simulink model "Gripper_Wrist_PID_check"  (R2019b)
settings: Solver=VariableStepAuto  StartTime=0.0  StopTime=10.0  FixedStep=0.0001  RelTol=1e-3
undefined symbols (not defined in the file): GR, WB, WJ, WKb, WKm, WL
libraries: cstblocks x2, simulink x1
settings Model: Creator=harsh  LastModifiedBy=harsh

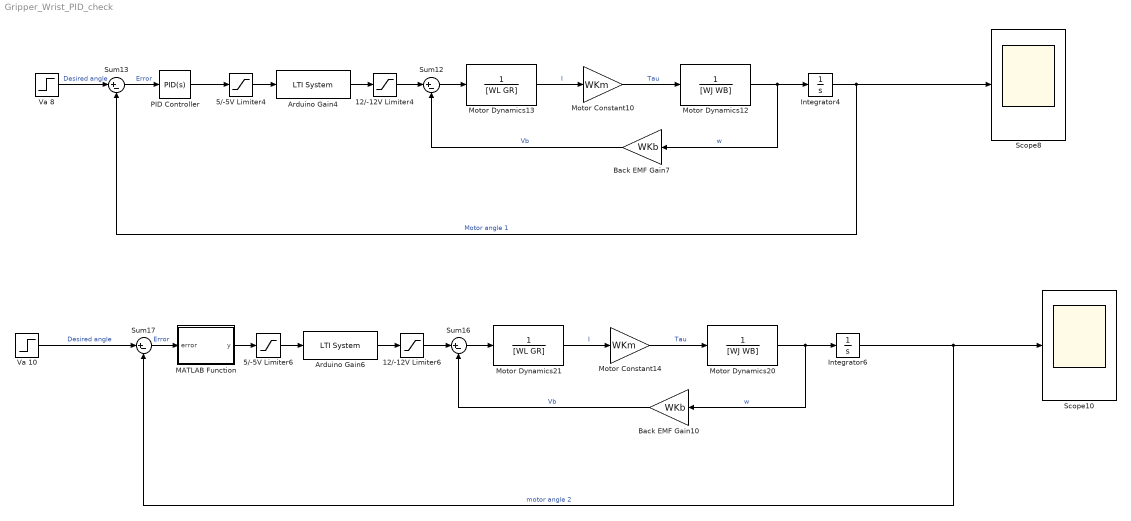
== system Gripper_Wrist_PID_check ==
  12/-12V Limiter4 : Saturate  UpperLimit=12  LowerLimit=-12
  12/-12V Limiter6 : Saturate  UpperLimit=12  LowerLimit=-12
  5/-5V Limiter4 : Saturate  UpperLimit=5  LowerLimit=-5
  5/-5V Limiter6 : Saturate  UpperLimit=5  LowerLimit=-5
  Arduino Gain4 : cstblocks/LTI System  sys=OPAMP  IC=[]
  Arduino Gain6 : cstblocks/LTI System  sys=OPAMP  IC=[]
  Back EMF Gain10 : Gain  Gain=WKb
  Back EMF Gain7 : Gain  Gain=WKb
  Integrator4 : Integrator
  Integrator6 : Integrator
  MATLAB Function : MATLAB Function  TreatAsAtomicUnit=on
  Motor Constant10 : Gain  Gain=WKm
  Motor Constant14 : Gain  Gain=WKm
  Motor Dynamics12 : TransferFcn  Denominator=[WJ WB]
  Motor Dynamics13 : TransferFcn  Denominator=[WL GR]
  Motor Dynamics20 : TransferFcn  Denominator=[WJ WB]
  Motor Dynamics21 : TransferFcn  Denominator=[WL GR]
  PID Controller : simulink/Continuous/PID Controller  Controller=PID  Form=Parallel  TimeDomain=Continuous-time  SampleTime=-1  IntegratorMethod=Forward Euler  FilterMethod=Forward Euler  ControllerParametersSource=internal  P=7.36971279377399  I=24.525158078184  D=0.0474430843490964  UseFilter=on  N=5000  TunerSelectOption=Transfer Function Based (PID Tuner App)  InitialConditionSource=internal  InitialConditionForIntegrator=0  InitialConditionForFilter=0  DifferentiatorICPrevScaledInput=0  ExternalReset=none  TrackingMode=off  Kt=1  LimitOutput=off  UpperSaturationLimit=inf  LowerSaturationLimit=-inf  LinearizeAsGain=on  AntiWindupMode=none  Kb=1  POutMin=[]  POutMax=[]  IOutMin=[]  IOutMax=[]  DOutMin=[]  DOutMax=[]  NOutMin=[]  NOutMax=[]  SumOutMin=[]  SumOutMax=[]  SaturationOutMin=[]  SaturationOutMax=[]  PParamMin=[]  PParamMax=[]  IParamMin=[]  IParamMax=[]  DParamMin=[]  DParamMax=[]  NParamMin=[]  NParamMax=[]  KbParamMin=[]  KbParamMax=[]  KtParamMin=[]  KtParamMax=[]  KbOutMin=[]  KbOutMax=[]  KtOutMin=[]  KtOutMax=[]  IntegratorOutMin=[]  IntegratorOutMax=[]  FilterOutMin=[]  FilterOutMax=[]  SumI1OutMin=[]  SumI1OutMax=[]  SumI2OutMin=[]  SumI2OutMax=[]  SumI3OutMin=[]  SumI3OutMax=[]  SumI4OutMin=[]  SumI4OutMax=[]  SumDOutMin=[]  SumDOutMax=[]  DifferentiatorOutMin=[]  DifferentiatorOutMax=[]  FilterDiffOutCoefMin=[]  FilterDiffOutCoefMax=[]  ReciprocalOutMin=[]  ReciprocalOutMax=[]  SumDenOutMin=[]  SumDenOutMax=[]  SumNumOutMin=[]  SumNumOutMax=[]  DivideOutMin=[]  DivideOutMax=[]  IntegratorContinuousStateAttributes=''  IntegratorStateMustResolveToSignalObject=off  IntegratorRTWStateStorageClass=Auto  FilterContinuousStateAttributes=''  FilterStateMustResolveToSignalObject=off  FilterRTWStateStorageClass=Auto  ParallelPVariant=InternalParameters  IdealPVariant=Disabled  IVariant=InternalParameters  DVariant=InternalParameters  IntegratorVariant=Continuous  SatVariant=Disabled  AWVariant=Passthrough  PCopyVariant=Disabled  TRVariant=Disabled  FdbkBlocksVariant=Forward  IdealPFdbkVariant=Disabled  SatFdbkVariant=Disabled  DerivativeFilterVariant=ContFilter  NVariant=InternalParameters  NCopyVariant=Disabled  FilterICVariant=InternalICsFilter  IntegratorICVariant=InternalICs  ExternalResetVariant=Disabled  TRSumVariant=Passthrough  SumFdbkVariant=Disabled  SumVariant=Sum_PID
  Scope10 : Scope
  Scope8 : Scope
  Sum{12..13,16..17} (4 alike) : Sum  Inputs=|+-
  Va 10 : Step  After=pi/2  SampleTime=0
  Va 8 : Step  After=pi/2  SampleTime=0
  wires:
  Integrator6/1 -> Sum17/2, Scope10/1  "motor angle 2"
  Motor Dynamics20/1 -> Back EMF Gain10/1, Integrator6/1  "w"
  Sum16/1 -> Motor Dynamics21/1
  12/-12V Limiter6/1 -> Sum16/1
  Motor Constant14/1 -> Motor Dynamics20/1  "Tau"
  Sum17/1 -> MATLAB Function/1(error)  "Error"
  Motor Dynamics21/1 -> Motor Constant14/1  "I"
  5/-5V Limiter4/1 -> Arduino Gain4/1
  Back EMF Gain10/1 -> Sum16/2  "Vb"
  Arduino Gain4/1 -> 12/-12V Limiter4/1
  Back EMF Gain7/1 -> Sum12/2  "Vb"
  Integrator4/1 -> Scope8/1, Sum13/2  "Motor angle 1"
  5/-5V Limiter6/1 -> Arduino Gain6/1
  Sum12/1 -> Motor Dynamics13/1
  12/-12V Limiter4/1 -> Sum12/1
  Motor Constant10/1 -> Motor Dynamics12/1  "Tau"
  Motor Dynamics12/1 -> Back EMF Gain7/1, Integrator4/1  "w"
  Va 8/1 -> Sum13/1  "Desired angle"
  Va 10/1 -> Sum17/1  "Desired angle"
  Arduino Gain6/1 -> 12/-12V Limiter6/1
  Motor Dynamics13/1 -> Motor Constant10/1  "I"
  MATLAB Function/1(y) -> 5/-5V Limiter6/1
  PID Controller/1 -> 5/-5V Limiter4/1
  Sum13/1 -> PID Controller/1  "Error"

== matlab function Gripper_Wrist_PID_check/MATLAB Function ==
  settings: updateMethod=DISCRETE  sampleTime=0.0001
  data: error input; y output
function y = fcn(error)

persistent previous_error;                  %previous error = current error for next iteration, initially set to 0;
persistent Ki_output;                        %need as persistent variable for Ki_output = Ki_output + (...)
persistent ept;                             %constant vector of exponentials (p*e^(-p*n*Ts)) where n = 1.....#of samples we want to average
persistent unweighted_differential_outputs;  %vector used for dot product with ept, shifted at each cycle. 

if isempty(previous_error)
    previous_error = 0;
end

%Trial values for testing against Built in PID block
Kp = 7.3697;
Ki = 24.525;
Kd = 0.04744;

Ts = 0.0001;    %Controller frequency from Arduino assumed to be 10kHz.

%--------P controller part------------------
Kp_output = Kp*error;    

%---------I controller part-----------------

%Initializing Ki_output
if isempty(Ki_output)
    Ki_output = 0;
end

Ki_output = Ki_output + Ki*[(error + previous_error)/2]*Ts; %cumulative areas of trapeziums

%----------D controller part----------------
controlfreq = 10000; %Hz
filter_pole = 5000;  %big pole because we don't care much about averaging but we do care a lot about delay. (signal is not noisy)
n = 4*controlfreq/filter_pole;  %We are averaging 80 samples in this example


%Now, we initialize the ept vector (will remain constant valued throughout the program)
if isempty(ept)
    ept = zeros(1,n);
    for i = 1:n
        ept(i) = filter_pole*1.132*exp(-filter_pole*i*Ts);
    end
    %We want Ts*sum(ept) = 1 but this is not the case normally, so we have to scale the ept such that we get a sum
    %of 1. To account for discretization error, we scale it by multiplying it by 1.132 in this example. 
end

if isempty(unweighted_differential_outputs)
    unweighted_differential_outputs = zeros(1,n);
end 

unweighted_differential_outputs(1) = (error - previous_error); 
filtered_derivative = dot(ept,unweighted_differential_outputs);

Kd_output = Kd*filtered_derivative;

n2 = n+1; %n2 = 9
for count = 1:(n-1) %1:7 in this example
    unweighted_differential_outputs(n2-count) = unweighted_differential_outputs(n2 - count - 1);    %shift values by one index, and in next loop calculate one more new slope at index 1 (starting index)
end 

y = Kp_output + Ki_output + Kd_output;

previous_error = error; %this will help us move on to get new values for Ki and Kd

end
